simulink model "aufgabe_7_sim"  (R2016b)
settings: Solver=VariableStepAuto  StartTime=0.0  StopTime=14  RelTol=1e-3
values from neighbouring files (symbols this model uses):
  M_ext_r = 0    [aufgabe_4.m]    (also in aufgabe_6.m)
  te = .05    (= 0.05)    [Esys_Parameter.m]    (also in aufgabe_1.m = 1; aufgabe_6.m = 1)
  ts = .1    (= 0.1)    [Esys_Parameter.m]    (also in aufgabe_1.m = 3; aufgabe_6.m = 0.5)
  u_GSM_r = 5.6    [aufgabe_4.m]    (also in aufgabe_6.m)
  Usinus = 1    [Esys_Parameter.m]    (also in aufgabe_1.m = 0.1; aufgabe_6.m)
  w_P_r = -(R_GSM*d_vP + R_GSM*d_vGSM - (k_GSM^4 + R_GSM^2*d_vP^2 +      R_GSM^2*d_vGSM^2 - 4*M_ext_r*R_GSM^2*d_qP -      4*R_GSM^2*d_cP*d_qP - 4*R_GSM^2*d_cGSM*d_qP +      2*R_GSM^2*d_vP*d_vGSM + 2*R_GSM*d_vP*k_GSM^2 +      2*R_GSM*d_vGSM*k_GSM^2 + 4*R_GSM*d_qP*k_GSM*u_GSM_r)^(1/2) +      k_GSM^2)/(2*R_GSM*d_qP)    [aufgabe_4.m]    (also in aufgabe_5.m = -(R_GSM*d_vP + R_GSM*d_vGSM - (k_GSM^4 + R_GSM^2*d_vP^2 +   ; aufgabe_6.m)
  we = 1000    [Esys_Parameter.m]    (also in aufgabe_1.m = 10; aufgabe_6.m = 2)
libraries: cstblocks x6, simulink x1
settings Model: Creator=M  LastModifiedBy=M

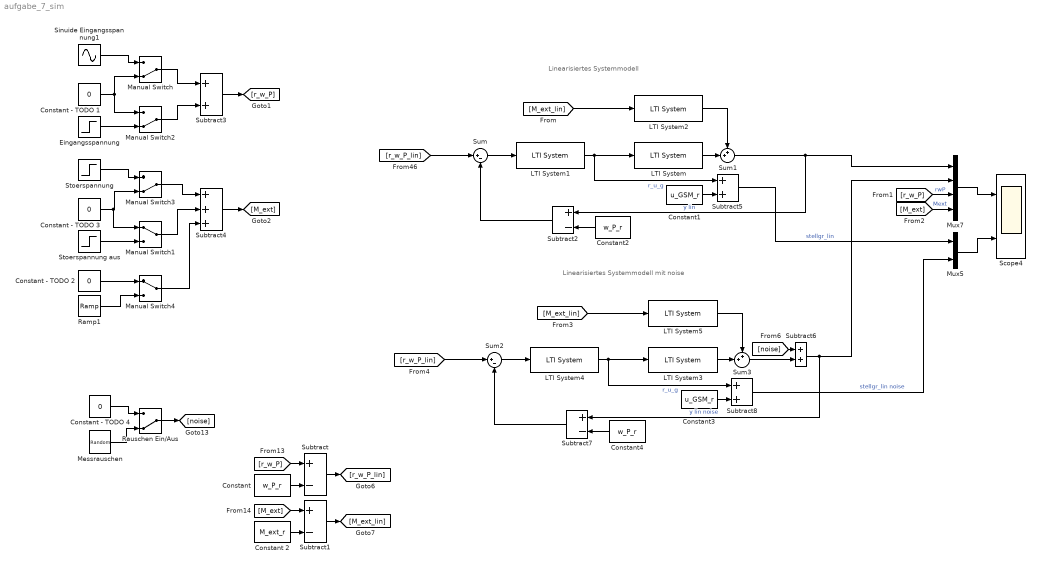
== system aufgabe_7_sim ==
  note: Linearisiertes Systemmodell
  note: Linearisiertes Systemmodell mit noise
  Constant : Constant  Value=w_P_r
  Constant - TODO {1..4} (4 alike) : Constant  Value=0
  Constant 2 : Constant  Value=M_ext_r
  Constant1 : Constant  Value=u_GSM_r
  Constant2 : Constant  Value=w_P_r
  Constant3 : Constant  Value=u_GSM_r
  Constant4 : Constant  Value=w_P_r
  Eingangsspannung : Step  Time=te  After=20  SampleTime=0
  LTI System : cstblocks/LTI System  sys=Gz_lin  IC=[]
  LTI System1 : cstblocks/LTI System  sys=Rz_tr4  IC=[]
  LTI System2 : cstblocks/LTI System  sys=Gzd_lin  IC=[]
  LTI System3 : cstblocks/LTI System  sys=Gz_lin  IC=[]
  LTI System4 : cstblocks/LTI System  sys=Rz_tr4  IC=[]
  LTI System5 : cstblocks/LTI System  sys=Gzd_lin  IC=[]
  Manual Switch : ManualSwitch  CurrentSetting=0
  Manual Switch1 : ManualSwitch
  Manual Switch2 : ManualSwitch  CurrentSetting=0
  Manual Switch3 : ManualSwitch  CurrentSetting=0
  Manual Switch4 : ManualSwitch
  Messrauschen : UniformRandomNumber  Minimum=-5e-2  Maximum=5e-2  SampleTime=1e-3
  Mux5 : Mux  Inputs=2
  Mux7 : Mux
  Ramp1 : simulink/Sources/Ramp  slope=1  start=tr  X0=0
  Rauschen Ein/Aus : ManualSwitch  CurrentSetting=0
  Scope4 : Scope  NumInputPorts=2
  Sinuide Eingangsspannung1 : Sin  Amplitude=Usinus  Bias=u_GSM_r  Frequency=we  SampleTime=0
  Stoerspannung : Step  Time=ts  SampleTime=0
  Stoerspannung aus : Step  Time=10  After=-1  SampleTime=0
  Subtract{,1..2,7} (4 alike) : Sum  Inputs=+-
  Subtract{3,5..6,8} (4 alike) : Sum
  Subtract4 : Sum  Inputs=+++
  Sum : Sum  Inputs=|+-
  Sum1 : Sum  Inputs=++|
  Sum2 : Sum  Inputs=|+-
  Sum3 : Sum  Inputs=++|
  wires:
  Subtract/1 -> [r_w_P_lin]
  [r_w_P] -> Subtract/1
  Subtract1/1 -> [M_ext_lin]
  Constant 2/1 -> Subtract1/2
  Sum/1 -> LTI System1/1
  [r_w_P_lin] -> Sum/1
  LTI System1/1 -> Subtract5/1, LTI System/1  "r_u_g"
  LTI System/1 -> Sum1/2
  [M_ext_lin] -> LTI System2/1
  Subtract2/1 -> Sum/2
  Sinuide Eingangsspannung1/1 -> Manual Switch/1
  Constant - TODO 1/1 -> Manual Switch/2, Manual Switch2/1
  Eingangsspannung/1 -> Manual Switch2/2
  Manual Switch/1 -> Subtract3/1
  Manual Switch2/1 -> Subtract3/2
  Subtract3/1 -> [r_w_P]
  Stoerspannung/1 -> Manual Switch3/1
  Constant - TODO 3/1 -> Manual Switch1/1, Manual Switch3/2
  Ramp1/1 -> Manual Switch4/2
  Manual Switch3/1 -> Subtract4/1
  Subtract4/1 -> [M_ext]
  Stoerspannung aus/1 -> Manual Switch1/2
  Constant - TODO 2/1 -> Manual Switch4/1
  Manual Switch1/1 -> Subtract4/2
  Subtract5/1 -> Mux5/1  "stellgr_lin"
  LTI System2/1 -> Sum1/1
  Constant1/1 -> Subtract5/2
  [M_ext] -> Subtract1/1
  Manual Switch4/1 -> Subtract4/3
  Constant2/1 -> Subtract2/2
  Mux7/1 -> Scope4/1
  Mux5/1 -> Scope4/2
  [r_w_P] -> Mux7/3  "rwP"
  [M_ext] -> Mux7/4  "Mext"
  Constant/1 -> Subtract/2
  Messrauschen/1 -> Rauschen Ein/Aus/2
  Constant - TODO 4/1 -> Rauschen Ein/Aus/1
  Rauschen Ein/Aus/1 -> [noise]
  Sum1/1 -> Subtract2/1, Mux7/1  "y lin"
  Sum2/1 -> LTI System4/1
  [r_w_P_lin] -> Sum2/1
  LTI System4/1 -> Subtract8/1, LTI System3/1  "r_u_g"
  LTI System3/1 -> Sum3/2
  [M_ext_lin] -> LTI System5/1
  Subtract7/1 -> Sum2/2
  LTI System5/1 -> Sum3/1
  Constant3/1 -> Subtract8/2
  Constant4/1 -> Subtract7/2
  [noise] -> Subtract6/1
  Sum3/1 -> Subtract6/2
  Subtract6/1 -> Subtract7/1, Mux7/2  "y lin noise"
  Subtract8/1 -> Mux5/2  "stellgr_lin noise"
